simulink subsystem "inverterIn"  (R2022b)
settings: Solver=VariableStepAuto  StartTime=0.0  StopTime=10.0  RelTol=1e-3
libraries: Raptor_lib x19
settings Model: Creator=serga  LastModifiedBy=serga

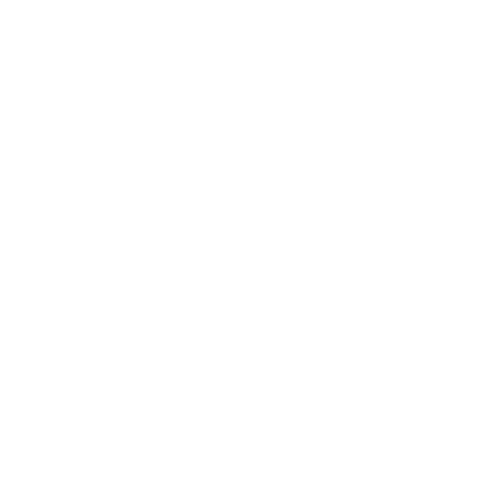
[thumbnail: Simulink's stored preview of the top-level diagram]
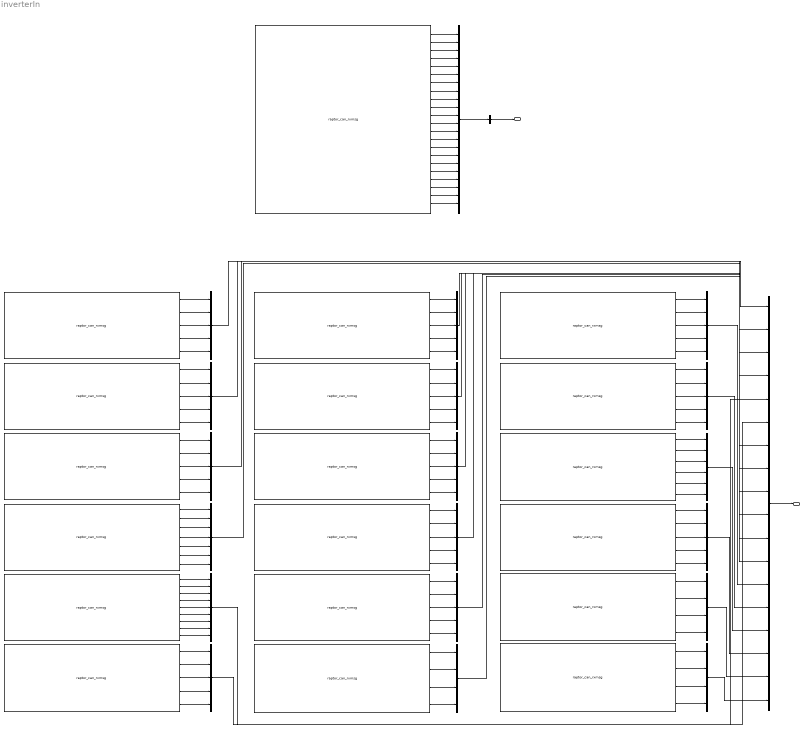
== system inverterIn ==
  note: CAN1
  note: CAN2
  Bus Creator : BusCreator  Inputs=22
  Bus Creator{1..3,6..11,13..14,16} (12 alike) : BusCreator  Inputs=5
  Bus Creator12 : BusCreator  Inputs=4
  Bus Creator15 : BusCreator  Inputs=6
  Bus Creator17 : BusCreator  Inputs=4
  Bus Creator18 : BusCreator  Inputs=4
  Bus Creator19 : BusCreator  Inputs=1
  Bus Creator20 : BusCreator  Inputs=18
  Bus Creator4 : BusCreator  Inputs=7
  Bus Creator5 : BusCreator  Inputs=9
  raptor_can_rxmsg1 : Raptor_lib/CAN/raptor_can_rxmsg  canDefinition=struct('dbcFile', 'raptor_CAN2.dbc','message', 'PM_161','comment', '','signals', {{'PM_controlBoardTemp','PM_rtd1Temp','PM_rtd2Temp','PM_rtd3Temp'}},'enabled', [ 1 1 1 1;],'scaled', [ 1 1 1 1;],'canBus', '''CAN2''','messageID', [ 161;],'idMask', [ 536870911;],'payloadMask', [],'payloadValue', [],'period', [ 0;],'mailbox', '''''','queueSize', [ 1;],'label', [ 1;],'ver', [ 2;],'showID', [ 0;],'showRaw', [ 0;],'showRawMsg', [ 0;],'useStartVals', [ 0;],'extendedId', [ 0;],'showAge', [ 1;],'useSimFunc', [ 0;],'sim_func_name', '''''','fill', [ 0;],'editID', [ 0;],'signalOrder', [ 1;],'signalAscDes', [ 1;],'msgLength', [ 8;])  canBus='CAN2'  mailbox=''  payloadMask=[]  payloadValue=[]  idMask=hex2dec('1FFFFFFF')  queueSize=1  showID=0  label=1  fill=0  id=161  showRaw=0  showAge=1  signalOrder=1  signalInfo={{struct('Name', 'PM_rtd3Temp','StartBit', [ 48;],'SignalSize', [ 16;],'ByteOrder', 'LittleEndian','ValueType', 'SIGNED','Class', 'int16','Signed', [ 1;],'Factor', [ 0.1;],'Offset', [ 0;],'Min', [ -3276.8;],'Max', [ 3276.7;],'Units', 'degC','StartVal', [ 0;],'Comment', 'RTD Input 3 (PT1000) Temperature (Gen 2 Only)','Multiplexed', [ 0;],'Multiplexor', [ 0;],'MultiplexMode_Min', [ 0;],'MultiplexMode_Max', [ 0;]),struct('Name', 'PM_rtd2Temp','StartBit', [ 32;],'SignalSize', [ 16;],'ByteOrder', 'LittleEndian','ValueType', 'SIGNED','Class', 'int16','Signed', [ 1;],'Factor', [ 0.1;],'Offset', [ 0;],'Min', [ -3276.8;],'Max', [ 3276.7;],'Units', 'degC','StartVal', [ 0;],'Comment', 'RTD Input 2 (PT1000) Temperature','Multiplexed', [ 0;],'Multiplexor', [ 0;],'MultiplexMode_Min', [ 0;],'MultiplexMode_Max', [ 0;]),struct('Name', 'PM_rtd1Temp','StartBit', [ 16;],'SignalSize', [ 16;],'ByteOrder', 'LittleEndian','ValueType', 'SIGNED','Class', 'int16','Signed', [ 1;],'Factor', [ 0.1;],'Offset', [ 0;],'Min', [ -3276.8;],'Max', [ 3276.7;],'Units', 'degC','StartVal', [ 0;],'Comment', 'RTD Input 1 (PT1000) Temperature','Multiplexed', [ 0;],'Multiplexor', [ 0;],'MultiplexMode_Min', [ 0;],'MultiplexMode_Max', [ 0;]),struct('Name', 'PM_controlBoardTemp','StartBit', [ 0;],'SignalSize', [ 16;],'ByteOrder', 'LittleEndian','ValueType', 'SIGNED','Class', 'int16','Signed', [ 1;],'Factor', [ 0.1;],'Offset', [ 0;],'Min', [ -3276.8;],'Max', [ 3276.7;],'Units', 'degC','StartVal', [ 0;],'Comment', 'Control Board Temperature','Multiplexed', [ 0;],'Multiplexor', [ 0;],'MultiplexMode_Min', [ 0;],'MultiplexMode_Max', [ 0;])}}  showRawMsg=0  useSimFunc=0  sim_func_name=''  useStartVals=0  extendedId=0
      settings: SourceProductName=Raptor
  raptor_can_rxmsg10 : Raptor_lib/CAN/raptor_can_rxmsg  canDefinition=struct('dbcFile', 'raptor_CAN2.dbc','message', 'PM_169','comment', '','signals', {{'PM_refVolt120','PM_refVolt15','PM_refVolt25','PM_refVolt50'}},'enabled', [ 1 1 1 1;],'scaled', [ 1 1 1 1;],'canBus', '''CAN2''','messageID', [ 169;],'idMask', [ 536870911;],'payloadMask', [],'payloadValue', [],'period', [ 0;],'mailbox', '''''','queueSize', [ 1;],'label', [ 1;],'ver', [ 2;],'showID', [ 0;],'showRaw', [ 0;],'showRawMsg', [ 0;],'useStartVals', [ 0;],'extendedId', [ 0;],'showAge', [ 1;],'useSimFunc', [ 0;],'sim_func_name', '''''','fill', [ 0;],'editID', [ 0;],'signalOrder', [ 1;],'signalAscDes', [ 1;],'msgLength', [ 8;])  canBus='CAN2'  mailbox=''  payloadMask=[]  payloadValue=[]  idMask=hex2dec('1FFFFFFF')  queueSize=1  showID=0  label=1  fill=0  id=169  showRaw=0  showAge=1  signalOrder=1  signalInfo={{struct('Name', 'PM_refVolt50','StartBit', [ 32;],'SignalSize', [ 16;],'ByteOrder', 'LittleEndian','ValueType', 'SIGNED','Class', 'int16','Signed', [ 1;],'Factor', [ 0.01;],'Offset', [ 0;],'Min', [ -327.68;],'Max', [ 327.67;],'Units', 'V','StartVal', [ 0;],'Comment', 'Transducer voltage','Multiplexed', [ 0;],'Multiplexor', [ 0;],'MultiplexMode_Min', [ 0;],'MultiplexMode_Max', [ 0;]),struct('Name', 'PM_refVolt25','StartBit', [ 16;],'SignalSize', [ 16;],'ByteOrder', 'LittleEndian','ValueType', 'SIGNED','Class', 'int16','Signed', [ 1;],'Factor', [ 0.01;],'Offset', [ 0;],'Min', [ -327.68;],'Max', [ 327.67;],'Units', 'V','StartVal', [ 0;],'Comment', 'Internal reference voltage','Multiplexed', [ 0;],'Multiplexor', [ 0;],'MultiplexMode_Min', [ 0;],'MultiplexMode_Max', [ 0;]),struct('Name', 'PM_refVolt15','StartBit', [ 0;],'SignalSize', [ 16;],'ByteOrder', 'LittleEndian','ValueType', 'SIGNED','Class', 'int16','Signed', [ 1;],'Factor', [ 0.01;],'Offset', [ 0;],'Min', [ -327.68;],'Max', [ 327.67;],'Units', 'V','StartVal', [ 0;],'Comment', 'Internal reference voltage','Multiplexed', [ 0;],'Multiplexor', [ 0;],'MultiplexMode_Min', [ 0;],'MultiplexMode_Max', [ 0;]),struct('Name', 'PM_refVolt120','StartBit', [ 48;],'SignalSize', [ 16;],'ByteOrder', 'LittleEndian','ValueType', 'SIGNED','Class', 'int16','Signed', [ 1;],'Factor', [ 0.01;],'Offset', [ 0;],'Min', [ -327.68;],'Max', [ 327.67;],'Units', 'V','StartVal', [ 0;],'Comment', '12V Input Voltage','Multiplexed', [ 0;],'Multiplexor', [ 0;],'MultiplexMode_Min', [ 0;],'MultiplexMode_Max', [ 0;])}}  showRawMsg=0  useSimFunc=0  sim_func_name=''  useStartVals=0  extendedId=0
      settings: SourceProductName=Raptor
  raptor_can_rxmsg11 : Raptor_lib/CAN/raptor_can_rxmsg  canDefinition=struct('dbcFile', 'raptor_CAN2.dbc','message', 'PM_171','comment', '','signals', {{'PM_postFaultHi','PM_postFaultLo','PM_runFaultHi','PM_runFaultLo'}},'enabled', [ 1 1 1 1;],'scaled', [ 1 1 1 1;],'canBus', '''CAN2''','messageID', [ 171;],'idMask', [ 536870911;],'payloadMask', [],'payloadValue', [],'period', [ 0;],'mailbox', '''''','queueSize', [ 1;],'label', [ 1;],'ver', [ 2;],'showID', [ 0;],'showRaw', [ 0;],'showRawMsg', [ 0;],'useStartVals', [ 0;],'extendedId', [ 0;],'showAge', [ 1;],'useSimFunc', [ 0;],'sim_func_name', '''''','fill', [ 0;],'editID', [ 0;],'signalOrder', [ 1;],'signalAscDes', [ 1;],'msgLength', [ 8;])  canBus='CAN2'  mailbox=''  payloadMask=[]  payloadValue=[]  idMask=hex2dec('1FFFFFFF')  queueSize=1  showID=0  label=1  fill=0  id=171  showRaw=0  showAge=1  signalOrder=1  signalInfo={{struct('Name', 'PM_runFaultLo','StartBit', [ 32;],'SignalSize', [ 16;],'ByteOrder', 'LittleEndian','ValueType', 'SIGNED','Class', 'int16','Signed', [ 1;],'Factor', [ 1;],'Offset', [ 0;],'Min', [ -32768;],'Max', [ 32767;],'Units', '','StartVal', [ 0;],'Comment', 'Each bit represents a fault. Please refer to PM100 Users Manual for details','Multiplexed', [ 0;],'Multiplexor', [ 0;],'MultiplexMode_Min', [ 0;],'MultiplexMode_Max', [ 0;]),struct('Name', 'PM_runFaultHi','StartBit', [ 48;],'SignalSize', [ 16;],'ByteOrder', 'LittleEndian','ValueType', 'SIGNED','Class', 'int16','Signed', [ 1;],'Factor', [ 1;],'Offset', [ 0;],'Min', [ -32768;],'Max', [ 32767;],'Units', '','StartVal', [ 0;],'Comment', 'Each bit represents a fault. Please refer to PM100 Users Manual for details','Multiplexed', [ 0;],'Multiplexor', [ 0;],'MultiplexMode_Min', [ 0;],'MultiplexMode_Max', [ 0;]),struct('Name', 'PM_postFaultLo','StartBit', [ 0;],'SignalSize', [ 16;],'ByteOrder', 'LittleEndian','ValueType', 'SIGNED','Class', 'int16','Signed', [ 1;],'Factor', [ 1;],'Offset', [ 0;],'Min', [ -32768;],'Max', [ 32767;],'Units', '','StartVal', [ 0;],'Comment', 'Each bit represents a fault. Please refer to PM100 Users Manual for details','Multiplexed', [ 0;],'Multiplexor', [ 0;],'MultiplexMode_Min', [ 0;],'MultiplexMode_Max', [ 0;]),struct('Name', 'PM_postFaultHi','StartBit', [ 16;],'SignalSize', [ 16;],'ByteOrder', 'LittleEndian','ValueType', 'SIGNED','Class', 'int16','Signed', [ 1;],'Factor', [ 1;],'Offset', [ 0;],'Min', [ -32768;],'Max', [ 32767;],'Units', '','StartVal', [ 0;],'Comment', 'Each bit represents a fault. Please refer to PM100 Users Manual for details','Multiplexed', [ 0;],'Multiplexor', [ 0;],'MultiplexMode_Min', [ 0;],'MultiplexMode_Max', [ 0;])}}  showRawMsg=0  useSimFunc=0  sim_func_name=''  useStartVals=0  extendedId=0
      settings: SourceProductName=Raptor
  raptor_can_rxmsg12 : Raptor_lib/CAN/raptor_can_rxmsg  canDefinition=struct('dbcFile', 'raptor_CAN2.dbc','message', 'PM_172','comment', '','signals', {{'PM_commandedTorque','PM_powerOnTimer','PM_torqueFeedback'}},'enabled', [ 1 1 1;],'scaled', [ 1 1 1;],'canBus', '''CAN2''','messageID', [ 172;],'idMask', [ 536870911;],'payloadMask', [],'payloadValue', [],'period', [ 0;],'mailbox', '''''','queueSize', [ 1;],'label', [ 1;],'ver', [ 2;],'showID', [ 0;],'showRaw', [ 0;],'showRawMsg', [ 0;],'useStartVals', [ 0;],'extendedId', [ 0;],'showAge', [ 1;],'useSimFunc', [ 0;],'sim_func_name', '''''','fill', [ 0;],'editID', [ 0;],'signalOrder', [ 1;],'signalAscDes', [ 1;],'msgLength', [ 8;])  canBus='CAN2'  mailbox=''  payloadMask=[]  payloadValue=[]  idMask=hex2dec('1FFFFFFF')  queueSize=1  showID=0  label=1  fill=0  id=172  showRaw=0  showAge=1  signalOrder=1  signalInfo={{struct('Name', 'PM_torqueFeedback','StartBit', [ 16;],'SignalSize', [ 16;],'ByteOrder', 'LittleEndian','ValueType', 'SIGNED','Class', 'int16','Signed', [ 1;],'Factor', [ 0.1;],'Offset', [ 0;],'Min', [ -3276.8;],'Max', [ 3276.7;],'Units', 'Nm','StartVal', [ 0;],'Comment', 'Estimated motor torque feedback','Multiplexed', [ 0;],'Multiplexor', [ 0;],'MultiplexMode_Min', [ 0;],'MultiplexMode_Max', [ 0;]),struct('Name', 'PM_powerOnTimer','StartBit', [ 32;],'SignalSize', [ 32;],'ByteOrder', 'LittleEndian','ValueType', 'UNSIGNED','Class', 'uint32','Signed', [ 0;],'Factor', [ 0.003;],'Offset', [ 0;],'Min', [ 0;],'Max', [ 12884800;],'Units', 'sec','StartVal', [ 0;],'Comment', 'Updated every 3 msec. This will roll over in approximately 150 days!','Multiplexed', [ 0;],'Multiplexor', [ 0;],'MultiplexMode_Min', [ 0;],'MultiplexMode_Max', [ 0;]),struct('Name', 'PM_commandedTorque','StartBit', [ 0;],'SignalSize', [ 16;],'ByteOrder', 'LittleEndian','ValueType', 'SIGNED','Class', 'int16','Signed', [ 1;],'Factor', [ 0.1;],'Offset', [ 0;],'Min', [ -3276.8;],'Max', [ 3276.7;],'Units', 'Nm','StartVal', [ 0;],'Comment', 'The commanded torque','Multiplexed', [ 0;],'Multiplexor', [ 0;],'MultiplexMode_Min', [ 0;],'MultiplexMode_Max', [ 0;])}}  showRawMsg=0  useSimFunc=0  sim_func_name=''  useStartVals=0  extendedId=0
      settings: SourceProductName=Raptor
  raptor_can_rxmsg13 : Raptor_lib/CAN/raptor_can_rxmsg  canDefinition=struct('dbcFile', 'raptor_CAN2.dbc','message', 'PM_173','comment', '','signals', {{'PM_fluxWeakeningOutput','PM_idCommand','PM_iqCommand','PM_modulationIndex'}},'enabled', [ 1 1 1 1;],'scaled', [ 1 1 1 1;],'canBus', '''CAN2''','messageID', [ 173;],'idMask', [ 536870911;],'payloadMask', [],'payloadValue', [],'period', [ 0;],'mailbox', '''''','queueSize', [ 1;],'label', [ 1;],'ver', [ 2;],'showID', [ 0;],'showRaw', [ 0;],'showRawMsg', [ 0;],'useStartVals', [ 0;],'extendedId', [ 0;],'showAge', [ 1;],'useSimFunc', [ 0;],'sim_func_name', '''''','fill', [ 0;],'editID', [ 0;],'signalOrder', [ 1;],'signalAscDes', [ 1;],'msgLength', [ 8;])  canBus='CAN2'  mailbox=''  payloadMask=[]  payloadValue=[]  idMask=hex2dec('1FFFFFFF')  queueSize=1  showID=0  label=1  fill=0  id=173  showRaw=0  showAge=1  signalOrder=1  signalInfo={{struct('Name', 'PM_modulationIndex','StartBit', [ 0;],'SignalSize', [ 16;],'ByteOrder', 'LittleEndian','ValueType', 'SIGNED','Class', 'int16','Signed', [ 1;],'Factor', [ 0.0001;],'Offset', [ 0;],'Min', [ -3.2768;],'Max', [ 3.2767;],'Units', '','StartVal', [ 0;],'Comment', 'This is the modulation index. The scale factor is x100. To get the actual modulation index divide value by 100','Multiplexed', [ 0;],'Multiplexor', [ 0;],'MultiplexMode_Min', [ 0;],'MultiplexMode_Max', [ 0;]),struct('Name', 'PM_iqCommand','StartBit', [ 48;],'SignalSize', [ 16;],'ByteOrder', 'LittleEndian','ValueType', 'SIGNED','Class', 'int16','Signed', [ 1;],'Factor', [ 0.1;],'Offset', [ 0;],'Min', [ -3276.8;],'Max', [ 3276.7;],'Units', 'A','StartVal', [ 0;],'Comment', 'The commanded Q-axis current','Multiplexed', [ 0;],'Multiplexor', [ 0;],'MultiplexMode_Min', [ 0;],'MultiplexMode_Max', [ 0;]),struct('Name', 'PM_idCommand','StartBit', [ 32;],'SignalSize', [ 16;],'ByteOrder', 'LittleEndian','ValueType', 'SIGNED','Class', 'int16','Signed', [ 1;],'Factor', [ 0.1;],'Offset', [ 0;],'Min', [ -3276.8;],'Max', [ 3276.7;],'Units', 'A','StartVal', [ 0;],'Comment', 'The commanded D-axis current','Multiplexed', [ 0;],'Multiplexor', [ 0;],'MultiplexMode_Min', [ 0;],'MultiplexMode_Max', [ 0;]),struct('Name', 'PM_fluxWeakeningOutput','StartBit', [ 16;],'SignalSize', [ 16;],'ByteOrder', 'LittleEndian','ValueType', 'SIGNED','Class', 'int16','Signed', [ 1;],'Factor', [ 0.1;],'Offset', [ 0;],'Min', [ -3276.8;],'Max', [ 3276.7;],'Units', 'A','StartVal', [ 0;],'Comment', 'This is the current output of the flux generator','Multiplexed', [ 0;],'Multiplexor', [ 0;],'MultiplexMode_Min', [ 0;],'MultiplexMode_Max', [ 0;])}}  showRawMsg=0  useSimFunc=0  sim_func_name=''  useStartVals=0  extendedId=0
      settings: SourceProductName=Raptor
  raptor_can_rxmsg14 : Raptor_lib/CAN/raptor_can_rxmsg  canDefinition=struct('dbcFile', 'raptor_CAN2.dbc','message', 'PM_174','comment', '','signals', {{'PM_datecodeMMDD','PM_datecodeYYYY','PM_projectCodeEEPVer','PM_swVersion'}},'enabled', [ 1 1 1 1;],'scaled', [ 1 1 1 1;],'canBus', '''CAN2''','messageID', [ 174;],'idMask', [ 536870911;],'payloadMask', [],'payloadValue', [],'period', [ 0;],'mailbox', '''''','queueSize', [ 1;],'label', [ 1;],'ver', [ 2;],'showID', [ 0;],'showRaw', [ 0;],'showRawMsg', [ 0;],'useStartVals', [ 0;],'extendedId', [ 0;],'showAge', [ 1;],'useSimFunc', [ 0;],'sim_func_name', '''''','fill', [ 0;],'editID', [ 0;],'signalOrder', [ 1;],'signalAscDes', [ 1;],'msgLength', [ 8;])  canBus='CAN2'  mailbox=''  payloadMask=[]  payloadValue=[]  idMask=hex2dec('1FFFFFFF')  queueSize=1  showID=0  label=1  fill=0  id=174  showRaw=0  showAge=1  signalOrder=1  signalInfo={{struct('Name', 'PM_swVersion','StartBit', [ 16;],'SignalSize', [ 16;],'ByteOrder', 'LittleEndian','ValueType', 'UNSIGNED','Class', 'uint16','Signed', [ 0;],'Factor', [ 1;],'Offset', [ 0;],'Min', [ 0;],'Max', [ 65535;],'Units', '','StartVal', [ 0;],'Comment', '','Multiplexed', [ 0;],'Multiplexor', [ 0;],'MultiplexMode_Min', [ 0;],'MultiplexMode_Max', [ 0;]),struct('Name', 'PM_projectCodeEEPVer','StartBit', [ 0;],'SignalSize', [ 16;],'ByteOrder', 'LittleEndian','ValueType', 'UNSIGNED','Class', 'uint16','Signed', [ 0;],'Factor', [ 1;],'Offset', [ 0;],'Min', [ 0;],'Max', [ 65535;],'Units', '','StartVal', [ 0;],'Comment', '','Multiplexed', [ 0;],'Multiplexor', [ 0;],'MultiplexMode_Min', [ 0;],'MultiplexMode_Max', [ 0;]),struct('Name', 'PM_datecodeYYYY','StartBit', [ 48;],'SignalSize', [ 16;],'ByteOrder', 'LittleEndian','ValueType', 'UNSIGNED','Class', 'uint16','Signed', [ 0;],'Factor', [ 1;],'Offset', [ 0;],'Min', [ 0;],'Max', [ 65535;],'Units', '','StartVal', [ 0;],'Comment', '','Multiplexed', [ 0;],'Multiplexor', [ 0;],'MultiplexMode_Min', [ 0;],'MultiplexMode_Max', [ 0;]),struct('Name', 'PM_datecodeMMDD','StartBit', [ 32;],'SignalSize', [ 16;],'ByteOrder', 'LittleEndian','ValueType', 'UNSIGNED','Class', 'uint16','Signed', [ 0;],'Factor', [ 1;],'Offset', [ 0;],'Min', [ 0;],'Max', [ 65535;],'Units', '','StartVal', [ 0;],'Comment', '','Multiplexed', [ 0;],'Multiplexor', [ 0;],'MultiplexMode_Min', [ 0;],'MultiplexMode_Max', [ 0;])}}  showRawMsg=0  useSimFunc=0  sim_func_name=''  useStartVals=0  extendedId=0
      settings: SourceProductName=Raptor
  raptor_can_rxmsg15 : Raptor_lib/CAN/raptor_can_rxmsg  canDefinition=struct('dbcFile', 'raptor_CAN2.dbc','message', 'PM_175','comment', '','signals', {{'PM_bufferRecord','PM_bufferSegment','PM_diagData1','PM_diagData2','PM_diagData3'}},'enabled', [ 1 1 1 1 1;],'scaled', [ 1 1 1 1 1;],'canBus', '''CAN2''','messageID', [ 175;],'idMask', [ 536870911;],'payloadMask', [],'payloadValue', [],'period', [ 0;],'mailbox', '''''','queueSize', [ 1;],'label', [ 1;],'ver', [ 2;],'showID', [ 0;],'showRaw', [ 0;],'showRawMsg', [ 0;],'useStartVals', [ 0;],'extendedId', [ 0;],'showAge', [ 1;],'useSimFunc', [ 0;],'sim_func_name', '''''','fill', [ 0;],'editID', [ 0;],'signalOrder', [ 1;],'signalAscDes', [ 1;],'msgLength', [ 8;])  canBus='CAN2'  mailbox=''  payloadMask=[]  payloadValue=[]  idMask=hex2dec('1FFFFFFF')  queueSize=1  showID=0  label=1  fill=0  id=175  showRaw=0  showAge=1  signalOrder=1  signalInfo={{struct('Name', 'PM_diagData3','StartBit', [ 48;],'SignalSize', [ 16;],'ByteOrder', 'LittleEndian','ValueType', 'SIGNED','Class', 'int16','Signed', [ 1;],'Factor', [ 1;],'Offset', [ 0;],'Min', [ -32768;],'Max', [ 32767;],'Units', '','StartVal', [ 0;],'Comment', '','Multiplexed', [ 0;],'Multiplexor', [ 0;],'MultiplexMode_Min', [ 0;],'MultiplexMode_Max', [ 0;]),struct('Name', 'PM_diagData2','StartBit', [ 32;],'SignalSize', [ 16;],'ByteOrder', 'LittleEndian','ValueType', 'SIGNED','Class', 'int16','Signed', [ 1;],'Factor', [ 1;],'Offset', [ 0;],'Min', [ -32768;],'Max', [ 32767;],'Units', '','StartVal', [ 0;],'Comment', '','Multiplexed', [ 0;],'Multiplexor', [ 0;],'MultiplexMode_Min', [ 0;],'MultiplexMode_Max', [ 0;]),struct('Name', 'PM_diagData1','StartBit', [ 16;],'SignalSize', [ 16;],'ByteOrder', 'LittleEndian','ValueType', 'SIGNED','Class', 'int16','Signed', [ 1;],'Factor', [ 1;],'Offset', [ 0;],'Min', [ -32768;],'Max', [ 32767;],'Units', '','StartVal', [ 0;],'Comment', '','Multiplexed', [ 0;],'Multiplexor', [ 0;],'MultiplexMode_Min', [ 0;],'MultiplexMode_Max', [ 0;]),struct('Name', 'PM_bufferSegment','StartBit', [ 8;],'SignalSize', [ 8;],'ByteOrder', 'LittleEndian','ValueType', 'UNSIGNED','Class', 'uint8','Signed', [ 0;],'Factor', [ 1;],'Offset', [ 0;],'Min', [ 0;],'Max', [ 5;],'Units', '','StartVal', [ 0;],'Comment', '','Multiplexed', [ 0;],'Multiplexor', [ 0;],'MultiplexMode_Min', [ 0;],'MultiplexMode_Max', [ 0;]),struct('Name', 'PM_bufferRecord','StartBit', [ 0;],'SignalSize', [ 8;],'ByteOrder', 'LittleEndian','ValueType', 'UNSIGNED','Class', 'uint8','Signed', [ 0;],'Factor', [ 1;],'Offset', [ 0;],'Min', [ 0;],'Max', [ 255;],'Units', '','StartVal', [ 0;],'Comment', '','Multiplexed', [ 0;],'Multiplexor', [ 0;],'MultiplexMode_Min', [ 0;],'MultiplexMode_Max', [ 0;])}}  showRawMsg=0  useSimFunc=0  sim_func_name=''  useStartVals=0  extendedId=0
      settings: SourceProductName=Raptor
  raptor_can_rxmsg16 : Raptor_lib/CAN/raptor_can_rxmsg  canDefinition=struct('dbcFile', 'raptor_CAN2.dbc','message', 'PM_176','comment', '','signals', {{'PM_fastDCBusVolt','PM_fastMotorSpeed','PM_fastTorqueCommand','PM_fastTorqueFeedback'}},'enabled', [ 1 1 1 1;],'scaled', [ 1 1 1 1;],'canBus', '''CAN2''','messageID', [ 176;],'idMask', [ 536870911;],'payloadMask', [],'payloadValue', [],'period', [ 0;],'mailbox', '''''','queueSize', [ 1;],'label', [ 1;],'ver', [ 2;],'showID', [ 0;],'showRaw', [ 0;],'showRawMsg', [ 0;],'useStartVals', [ 0;],'extendedId', [ 0;],'showAge', [ 1;],'useSimFunc', [ 0;],'sim_func_name', '''''','fill', [ 0;],'editID', [ 0;],'signalOrder', [ 1;],'signalAscDes', [ 1;],'msgLength', [ 8;])  canBus='CAN2'  mailbox=''  payloadMask=[]  payloadValue=[]  idMask=hex2dec('1FFFFFFF')  queueSize=1  showID=0  label=1  fill=0  id=176  showRaw=0  showAge=1  signalOrder=1  signalInfo={{struct('Name', 'PM_fastTorqueFeedback','StartBit', [ 16;],'SignalSize', [ 16;],'ByteOrder', 'LittleEndian','ValueType', 'SIGNED','Class', 'int16','Signed', [ 1;],'Factor', [ 0.1;],'Offset', [ 0;],'Min', [ -3276.8;],'Max', [ 3276.7;],'Units', 'Nm','StartVal', [ 0;],'Comment', 'The estimated torque','Multiplexed', [ 0;],'Multiplexor', [ 0;],'MultiplexMode_Min', [ 0;],'MultiplexMode_Max', [ 0;]),struct('Name', 'PM_fastTorqueCommand','StartBit', [ 0;],'SignalSize', [ 16;],'ByteOrder', 'LittleEndian','ValueType', 'SIGNED','Class', 'int16','Signed', [ 1;],'Factor', [ 0.1;],'Offset', [ 0;],'Min', [ -3276.8;],'Max', [ 3276.7;],'Units', 'Nm','StartVal', [ 0;],'Comment', 'The commanded torque','Multiplexed', [ 0;],'Multiplexor', [ 0;],'MultiplexMode_Min', [ 0;],'MultiplexMode_Max', [ 0;]),struct('Name', 'PM_fastMotorSpeed','StartBit', [ 32;],'SignalSize', [ 16;],'ByteOrder', 'LittleEndian','ValueType', 'SIGNED','Class', 'int16','Signed', [ 1;],'Factor', [ 1;],'Offset', [ 0;],'Min', [ -32768;],'Max', [ 32767;],'Units', 'rpm','StartVal', [ 0;],'Comment', 'Motor speed','Multiplexed', [ 0;],'Multiplexor', [ 0;],'MultiplexMode_Min', [ 0;],'MultiplexMode_Max', [ 0;]),struct('Name', 'PM_fastDCBusVolt','StartBit', [ 48;],'SignalSize', [ 16;],'ByteOrder', 'LittleEndian','ValueType', 'SIGNED','Class', 'int16','Signed', [ 1;],'Factor', [ 0.1;],'Offset', [ 0;],'Min', [ -3276.8;],'Max', [ 3276.7;],'Units', 'V','StartVal', [ 0;],'Comment', 'DC bus voltage','Multiplexed', [ 0;],'Multiplexor', [ 0;],'MultiplexMode_Min', [ 0;],'MultiplexMode_Max', [ 0;])}}  showRawMsg=0  useSimFunc=0  sim_func_name=''  useStartVals=0  extendedId=0
      settings: SourceProductName=Raptor
  raptor_can_rxmsg17 : Raptor_lib/CAN/raptor_can_rxmsg  canDefinition=struct('dbcFile', 'raptor_CAN2.dbc','message', 'PM_193','comment', '','signals', {{'PM_dataCommand','PM_parameterAddressCommand','PM_readWriteCommand'}},'enabled', [ 1 1 1;],'scaled', [ 1 1 1;],'canBus', '''CAN2''','messageID', [ 193;],'idMask', [ 536870911;],'payloadMask', [],'payloadValue', [],'period', [ 0;],'mailbox', '''''','queueSize', [ 1;],'label', [ 1;],'ver', [ 2;],'showID', [ 0;],'showRaw', [ 0;],'showRawMsg', [ 0;],'useStartVals', [ 0;],'extendedId', [ 0;],'showAge', [ 1;],'useSimFunc', [ 0;],'sim_func_name', '''''','fill', [ 0;],'editID', [ 0;],'signalOrder', [ 1;],'signalAscDes', [ 1;],'msgLength', [ 8;])  canBus='CAN2'  mailbox=''  payloadMask=[]  payloadValue=[]  idMask=hex2dec('1FFFFFFF')  queueSize=1  showID=0  label=1  fill=0  id=193  showRaw=0  showAge=1  signalOrder=1  signalInfo={{struct('Name', 'PM_readWriteCommand','StartBit', [ 16;],'SignalSize', [ 1;],'ByteOrder', 'LittleEndian','ValueType', 'UNSIGNED','Class', 'uint8','Signed', [ 0;],'Factor', [ 1;],'Offset', [ 0;],'Min', [ 0;],'Max', [ 1;],'Units', '','StartVal', [ 0;],'Comment', '0 = Read, 1 = Write','Multiplexed', [ 0;],'Multiplexor', [ 0;],'MultiplexMode_Min', [ 0;],'MultiplexMode_Max', [ 0;]),struct('Name', 'PM_parameterAddressCommand','StartBit', [ 0;],'SignalSize', [ 16;],'ByteOrder', 'LittleEndian','ValueType', 'UNSIGNED','Class', 'uint16','Signed', [ 0;],'Factor', [ 1;],'Offset', [ 0;],'Min', [ 0;],'Max', [ 65535;],'Units', '','StartVal', [ 0;],'Comment', 'Valid EEPROM Parameter CAN addresses are between 100 and 499','Multiplexed', [ 0;],'Multiplexor', [ 0;],'MultiplexMode_Min', [ 0;],'MultiplexMode_Max', [ 0;]),struct('Name', 'PM_dataCommand','StartBit', [ 32;],'SignalSize', [ 16;],'ByteOrder', 'LittleEndian','ValueType', 'SIGNED','Class', 'int16','Signed', [ 1;],'Factor', [ 1;],'Offset', [ 0;],'Min', [ -32768;],'Max', [ 32767;],'Units', '','StartVal', [ 0;],'Comment', 'All EEPROM data is 16 bits and is contained in bytes 4 and 5','Multiplexed', [ 0;],'Multiplexor', [ 0;],'MultiplexMode_Min', [ 0;],'MultiplexMode_Max', [ 0;])}}  showRawMsg=0  useSimFunc=0  sim_func_name=''  useStartVals=0  extendedId=0
      settings: SourceProductName=Raptor
  raptor_can_rxmsg18 : Raptor_lib/CAN/raptor_can_rxmsg  canDefinition=struct('dbcFile', 'raptor_CAN2.dbc','message', 'PM_194','comment', '','signals', {{'PM_dataResponse','PM_parameterAddressResponse','PM_writeSuccess'}},'enabled', [ 1 1 1;],'scaled', [ 1 1 1;],'canBus', '''CAN2''','messageID', [ 194;],'idMask', [ 536870911;],'payloadMask', [],'payloadValue', [],'period', [ 0;],'mailbox', '''''','queueSize', [ 1;],'label', [ 1;],'ver', [ 2;],'showID', [ 0;],'showRaw', [ 0;],'showRawMsg', [ 0;],'useStartVals', [ 0;],'extendedId', [ 0;],'showAge', [ 1;],'useSimFunc', [ 0;],'sim_func_name', '''''','fill', [ 0;],'editID', [ 0;],'signalOrder', [ 1;],'signalAscDes', [ 1;],'msgLength', [ 8;])  canBus='CAN2'  mailbox=''  payloadMask=[]  payloadValue=[]  idMask=hex2dec('1FFFFFFF')  queueSize=1  showID=0  label=1  fill=0  id=194  showRaw=0  showAge=1  signalOrder=1  signalInfo={{struct('Name', 'PM_writeSuccess','StartBit', [ 16;],'SignalSize', [ 1;],'ByteOrder', 'LittleEndian','ValueType', 'UNSIGNED','Class', 'uint8','Signed', [ 0;],'Factor', [ 1;],'Offset', [ 0;],'Min', [ 0;],'Max', [ 1;],'Units', '','StartVal', [ 0;],'Comment', '0 = Write Failure, 1 = Success','Multiplexed', [ 0;],'Multiplexor', [ 0;],'MultiplexMode_Min', [ 0;],'MultiplexMode_Max', [ 0;]),struct('Name', 'PM_parameterAddressResponse','StartBit', [ 0;],'SignalSize', [ 16;],'ByteOrder', 'LittleEndian','ValueType', 'UNSIGNED','Class', 'uint16','Signed', [ 0;],'Factor', [ 1;],'Offset', [ 0;],'Min', [ 0;],'Max', [ 65535;],'Units', '','StartVal', [ 0;],'Comment', 'Valid EEPROM Parameter CAN addresses are between 100 and 499','Multiplexed', [ 0;],'Multiplexor', [ 0;],'MultiplexMode_Min', [ 0;],'MultiplexMode_Max', [ 0;]),struct('Name', 'PM_dataResponse','StartBit', [ 32;],'SignalSize', [ 16;],'ByteOrder', 'LittleEndian','ValueType', 'SIGNED','Class', 'int16','Signed', [ 1;],'Factor', [ 1;],'Offset', [ 0;],'Min', [ -32768;],'Max', [ 32767;],'Units', '','StartVal', [ 0;],'Comment', 'All EEPROM data is 16 bits and is contained in bytes 4 and 5. Bytes 6 and 7 should be ignored','Multiplexed', [ 0;],'Multiplexor', [ 0;],'MultiplexMode_Min', [ 0;],'MultiplexMode_Max', [ 0;])}}  showRawMsg=0  useSimFunc=0  sim_func_name=''  useStartVals=0  extendedId=0
      settings: SourceProductName=Raptor
  raptor_can_rxmsg19 : Raptor_lib/CAN/raptor_can_rxmsg  canDefinition=struct('dbcFile', 'raptor_CAN1.dbc','message', 'PM_170','comment', '','signals', {{'PM_bmsActive','PM_bmsTorqueLimiting','PM_counterMsg170','PM_directionCommand','PM_inverterCommandMode','PM_inverterDischargeMode','PM_inverterEnableLockout','PM_inverterEnableState','PM_inverterRunMode','PM_inverterState','PM_lowSpeedLimiting','PM_maxSpeedLimiting','PM_pwmFrequency','PM_relayStatus1','PM_relayStatus2','PM_relayStatus3','PM_relayStatus4','PM_relayStatus5','PM_relayStatus6','PM_startModeActive','PM_vsmState'}},'enabled', [ 1 1 1 1 1 1 1 1 1 1 1 1 1 1 1 1 1 1 1 1 1;],'scaled', [ 1 1 1 1 1 1 1 1 1 1 1 1 1 1 1 1 1 1 1 1 1;],'canBus', '''CAN1''','messageID', [ 170;],'idMask', [ 536870911;],'payloadMask', [],'payloadValue', [],'period', [ 0;],'mailbox', '''''','queueSize', [ 1;],'label', [ 1;],'ver', [ 2;],'showID', [ 0;],'showRaw', [ 0;],'showRawMsg', [ 0;],'useStartVals', [ 0;],'extendedId', [ 0;],'showAge', [ 1;],'useSimFunc', [ 0;],'sim_func_name', '''''','fill', [ 0;],'editID', [ 0;],'signalOrder', [ 1;],'signalAscDes', [ 1;],'msgLength', [ 8;])  canBus='CAN1'  mailbox=''  payloadMask=[]  payloadValue=[]  idMask=hex2dec('1FFFFFFF')  queueSize=1  showID=0  label=1  fill=0  id=170  showRaw=0  showAge=1  signalOrder=1  signalInfo={{struct('Name', 'PM_vsmState','StartBit', [ 0;],'SignalSize', [ 8;],'ByteOrder', 'LittleEndian','ValueType', 'UNSIGNED','Class', 'uint8','Signed', [ 0;],'Factor', [ 1;],'Offset', [ 0;],'Min', [ 0;],'Max', [ 15;],'Units', '','StartVal', [ 0;],'Comment', 'Different states for the vehicle state machine','Multiplexed', [ 0;],'Multiplexor', [ 0;],'MultiplexMode_Min', [ 0;],'MultiplexMode_Max', [ 0;]),struct('Name', 'PM_startModeActive','StartBit', [ 54;],'SignalSize', [ 1;],'ByteOrder', 'LittleEndian','ValueType', 'UNSIGNED','Class', 'uint8','Signed', [ 0;],'Factor', [ 1;],'Offset', [ 0;],'Min', [ 0;],'Max', [ 1;],'Units', '','StartVal', [ 0;],'Comment', 'If in Key Switch Mode 1, indicates status of Start input being applied. 0 = Not Active, 1 = Active','Multiplexed', [ 0;],'Multiplexor', [ 0;],'MultiplexMode_Min', [ 0;],'MultiplexMode_Max', [ 0;]),struct('Name', 'PM_relayStatus6','StartBit', [ 29;],'SignalSize', [ 1;],'ByteOrder', 'LittleEndian','ValueType', 'UNSIGNED','Class', 'uint8','Signed', [ 0;],'Factor', [ 1;],'Offset', [ 0;],'Min', [ 0;],'Max', [ 1;],'Units', '','StartVal', [ 0;],'Comment', '0 = OFF, 1 = ON','Multiplexed', [ 0;],'Multiplexor', [ 0;],'MultiplexMode_Min', [ 0;],'MultiplexMode_Max', [ 0;]),struct('Name', 'PM_relayStatus5','StartBit', [ 28;],'SignalSize', [ 1;],'ByteOrder', 'LittleEndian','ValueType', 'UNSIGNED','Class', 'uint8','Signed', [ 0;],'Factor', [ 1;],'Offset', [ 0;],'Min', [ 0;],'Max', [ 1;],'Units', '','StartVal', [ 0;],'Comment', '0 = OFF, 1 = ON','Multiplexed', [ 0;],'Multiplexor', [ 0;],'MultiplexMode_Min', [ 0;],'MultiplexMode_Max', [ 0;]),struct('Name', 'PM_relayStatus4','StartBit', [ 27;],'SignalSize', [ 1;],'ByteOrder', 'LittleEndian','ValueType', 'UNSIGNED','Class', 'uint8','Signed', [ 0;],'Factor', [ 1;],'Offset', [ 0;],'Min', [ 0;],'Max', [ 1;],'Units', '','StartVal', [ 0;],'Comment', '0 = OFF, 1 = ON','Multiplexed', [ 0;],'Multiplexor', [ 0;],'MultiplexMode_Min', [ 0;],'MultiplexMode_Max', [ 0;]),struct('Name', 'PM_relayStatus3','StartBit', [ 26;],'SignalSize', [ 1;],'ByteOrder', 'LittleEndian','ValueType', 'UNSIGNED','Class', 'uint8','Signed', [ 0;],'Factor', [ 1;],'Offset', [ 0;],'Min', [ 0;],'Max', [ 1;],'Units', '','StartVal', [ 0;],'Comment', '0 = OFF, 1 = ON','Multiplexed', [ 0;],'Multiplexor', [ 0;],'MultiplexMode_Min', [ 0;],'MultiplexMode_Max', [ 0;]),struct('Name', 'PM_relayStatus2','StartBit', [ 25;],'SignalSize', [ 1;],'ByteOrder', 'LittleEndian','ValueType', 'UNSIGNED','Class', 'uint8','Signed', [ 0;],'Factor', [ 1;],'Offset', [ 0;],'Min', [ 0;],'Max', [ 1;],'Units', '','StartVal', [ 0;],'Comment', '0 = OFF, 1 = ON','Multiplexed', [ 0;],'Multiplexor', [ 0;],'MultiplexMode_Min', [ 0;],'MultiplexMode_Max', [ 0;]),struct('Name', 'PM_relayStatus1','StartBit', [ 24;],'SignalSize', [ 1;],'ByteOrder', 'LittleEndian','ValueType', 'UNSIGNED','Class', 'uint8','Signed', [ 0;],'Factor', [ 1;],'Offset', [ 0;],'Min', [ 0;],'Max', [ 1;],'Units', '','StartVal', [ 0;],'Comment', '0 = OFF, 1 = ON','Multiplexed', [ 0;],'Multiplexor', [ 0;],'MultiplexMode_Min', [ 0;],'MultiplexMode_Max', [ 0;]),struct('Name', 'PM_pwmFrequency','StartBit', [ 8;],'SignalSize', [ 8;],'ByteOrder', 'LittleEndian','ValueType', 'UNSIGNED','Class', 'uint8','Signed', [ 0;],'Factor', [ 1;],'Offset', [ 0;],'Min', [ 0;],'Max', [ 255;],'Units', 'kHz','StartVal', [ 0;],'Comment', 'The inverter PWM frequency','Multiplexed', [ 0;],'Multiplexor', [ 0;],'MultiplexMode_Min', [ 0;],'MultiplexMode_Max', [ 0;]),struct('Name', 'PM_maxSpeedLimiting','StartBit', [ 59;],'SignalSize', [ 1;],'ByteOrder', 'LittleEndian','ValueType', 'UNSIGNED','Class', 'uint8','Signed', [ 0;],'Factor', [ 1;],'Offset', [ 0;],'Min', [ 0;],'Max', [ 1;],'Units', '','StartVal', [ 0;],'Comment', '0 = Not Limiting, 1 = Torque Limiting due to Maximum Speed','Multiplexed', [ 0;],'Multiplexor', [ 0;],'MultiplexMode_Min', [ 0;],'MultiplexMode_Max', [ 0;]),struct('Name', 'PM_lowSpeedLimiting','StartBit', [ 61;],'SignalSize', [ 1;],'ByteOrder', 'LittleEndian','ValueType', 'UNSIGNED','Class', 'uint8','Signed', [ 0;],'Factor', [ 1;],'Offset', [ 0;],'Min', [ 0;],'Max', [ 1;],'Units', '','StartVal', [ 0;],'Comment', '0 = Not Limiting, 1 = Current Limiting due to Low Motor Speed','Multiplexed', [ 0;],'Multiplexor', [ 0;],'MultiplexMode_Min', [ 0;],'MultiplexMode_Max', [ 0;]),struct('Name', 'PM_inverterState','StartBit', [ 16;],'SignalSize', [ 8;],'ByteOrder', 'LittleEndian','ValueType', 'UNSIGNED','Class', 'uint8','Signed', [ 0;],'Factor', [ 1;],'Offset', [ 0;],'Min', [ 0;],'Max', [ 255;],'Units', '','StartVal', [ 0;],'Comment', 'Different states for the inverter machine state','Multiplexed', [ 0;],'Multiplexor', [ 0;],'MultiplexMode_Min', [ 0;],'MultiplexMode_Max', [ 0;]),struct('Name', 'PM_inverterRunMode','StartBit', [ 32;],'SignalSize', [ 1;],'ByteOrder', 'LittleEndian','ValueType', 'UNSIGNED','Class', 'uint8','Signed', [ 0;],'Factor', [ 1;],'Offset', [ 0;],'Min', [ 0;],'Max', [ 1;],'Units', '','StartVal', [ 0;],'Comment', '0 = Torque Mode, 1 = Speed Mode','Multiplexed', [ 0;],'Multiplexor', [ 0;],'MultiplexMode_Min', [ 0;],'MultiplexMode_Max', [ 0;]),struct('Name', 'PM_inverterEnableState','StartBit', [ 48;],'SignalSize', [ 1;],'ByteOrder', 'LittleEndian','ValueType', 'UNSIGNED','Class', 'uint8','Signed', [ 0;],'Factor', [ 1;],'Offset', [ 0;],'Min', [ 0;],'Max', [ 1;],'Units', '','StartVal', [ 0;],'Comment', '0 = Inverter Disabled, 1 = Inverter Enabled','Multiplexed', [ 0;],'Multiplexor', [ 0;],'MultiplexMode_Min', [ 0;],'MultiplexMode_Max', [ 0;]),struct('Name', 'PM_inverterEnableLockout','StartBit', [ 55;],'SignalSize', [ 1;],'ByteOrder', 'LittleEndian','ValueType', 'UNSIGNED','Class', 'uint8','Signed', [ 0;],'Factor', [ 1;],'Offset', [ 0;],'Min', [ 0;],'Max', [ 1;],'Units', '','StartVal', [ 0;],'Comment', '0 = Lockout Disabled, 1 = Lockout Enabled','Multiplexed', [ 0;],'Multiplexor', [ 0;],'MultiplexMode_Min', [ 0;],'MultiplexMode_Max', [ 0;]),struct('Name', 'PM_inverterDischargeMode','StartBit', [ 37;],'SignalSize', [ 3;],'ByteOrder', 'LittleEndian','ValueType', 'UNSIGNED','Class', 'uint8','Signed', [ 0;],'Factor', [ 1;],'Offset', [ 0;],'Min', [ 0;],'Max', [ 7;],'Units', '','StartVal', [ 0;],'Comment', '0 = Disabled, 1 = Enabled, 2 = Speed Check, 3 = Active, 4 = Complete','Multiplexed', [ 0;],'Multiplexor', [ 0;],'MultiplexMode_Min', [ 0;],'MultiplexMode_Max', [ 0;]),struct('Name', 'PM_inverterCommandMode','StartBit', [ 40;],'SignalSize', [ 1;],'ByteOrder', 'LittleEndian','ValueType', 'UNSIGNED','Class', 'uint8','Signed', [ 0;],'Factor', [ 1;],'Offset', [ 0;],'Min', [ 0;],'Max', [ 1;],'Units', '','StartVal', [ 0;],'Comment', '0 = CAN Mode, 1 = VSM Mode','Multiplexed', [ 0;],'Multiplexor', [ 0;],'MultiplexMode_Min', [ 0;],'MultiplexMode_Max', [ 0;]),struct('Name', 'PM_directionCommand','StartBit', [ 56;],'SignalSize', [ 1;],'ByteOrder', 'LittleEndian','ValueType', 'UNSIGNED','Class', 'uint8','Signed', [ 0;],'Factor', [ 1;],'Offset', [ 0;],'Min', [ 0;],'Max', [ 1;],'Units', '','StartVal', [ 0;],'Comment', '1 = Forward, 0 = `Reverse` if inverter enabled & `Stopped` if inverter is disabled','Multiplexed', [ 0;],'Multiplexor', [ 0;],'MultiplexMode_Min', [ 0;],'MultiplexMode_Max', [ 0;]),struct('Name', 'PM_counterMsg170','StartBit', [ 44;],'SignalSize', [ 4;],'ByteOrder', 'LittleEndian','ValueType', 'UNSIGNED','Class', 'uint8','Signed', [ 0;],'Factor', [ 1;],'Offset', [ 0;],'Min', [ 0;],'Max', [ 15;],'Units', '','StartVal', [ 0;],'Comment', 'Counter Message 170','Multiplexed', [ 0;],'Multiplexor', [ 0;],'MultiplexMode_Min', [ 0;],'MultiplexMode_Max', [ 0;]),struct('Name', 'PM_bmsTorqueLimiting','StartBit', [ 58;],'SignalSize', [ 1;],'ByteOrder', 'LittleEndian','ValueType', 'UNSIGNED','Class', 'uint8','Signed', [ 0;],'Factor', [ 1;],'Offset', [ 0;],'Min', [ 0;],'Max', [ 1;],'Units', '','StartVal', [ 0;],'Comment', '0 = Not Limiting, 1 = Limiting','Multiplexed', [ 0;],'Multiplexor', [ 0;],'MultiplexMode_Min', [ 0;],'MultiplexMode_Max', [ 0;]),struct('Name', 'PM_bmsActive','StartBit', [ 57;],'SignalSize', [ 1;],'ByteOrder', 'LittleEndian','ValueType', 'UNSIGNED','Class', 'uint8','Signed', [ 0;],'Factor', [ 1;],'Offset', [ 0;],'Min', [ 0;],'Max', [ 1;],'Units', '','StartVal', [ 0;],'Comment', '0 = BMS Not Active, 1 = BMS Active','Multiplexed', [ 0;],'Multiplexor', [ 0;],'MultiplexMode_Min', [ 0;],'MultiplexMode_Max', [ 0;])}}  showRawMsg=0  useSimFunc=0  sim_func_name=''  useStartVals=0  extendedId=0
      settings: SourceProductName=Raptor
  raptor_can_rxmsg2 : Raptor_lib/CAN/raptor_can_rxmsg  canDefinition=struct('dbcFile', 'raptor_CAN2.dbc','message', 'PM_160','comment', '','signals', {{'PM_gateDriverBoard','PM_moduleATemp','PM_moduleBTemp','PM_moduleCTemp'}},'enabled', [ 1 1 1 1;],'scaled', [ 1 1 1 1;],'canBus', '''CAN2''','messageID', [ 160;],'idMask', [ 536870911;],'payloadMask', [],'payloadValue', [],'period', [ 0;],'mailbox', '''''','queueSize', [ 1;],'label', [ 1;],'ver', [ 2;],'showID', [ 0;],'showRaw', [ 0;],'showRawMsg', [ 0;],'useStartVals', [ 0;],'extendedId', [ 0;],'showAge', [ 1;],'useSimFunc', [ 0;],'sim_func_name', '''''','fill', [ 0;],'editID', [ 0;],'signalOrder', [ 1;],'signalAscDes', [ 1;],'msgLength', [ 8;])  canBus='CAN2'  mailbox=''  payloadMask=[]  payloadValue=[]  idMask=hex2dec('1FFFFFFF')  queueSize=1  showID=0  label=1  fill=0  id=160  showRaw=0  showAge=1  signalOrder=1  signalInfo={{struct('Name', 'PM_moduleCTemp','StartBit', [ 32;],'SignalSize', [ 16;],'ByteOrder', 'LittleEndian','ValueType', 'SIGNED','Class', 'int16','Signed', [ 1;],'Factor', [ 0.1;],'Offset', [ 0;],'Min', [ -3276.8;],'Max', [ 3276.7;],'Units', 'degC','StartVal', [ 0;],'Comment', 'IGBT Module C Temperature','Multiplexed', [ 0;],'Multiplexor', [ 0;],'MultiplexMode_Min', [ 0;],'MultiplexMode_Max', [ 0;]),struct('Name', 'PM_moduleBTemp','StartBit', [ 16;],'SignalSize', [ 16;],'ByteOrder', 'LittleEndian','ValueType', 'SIGNED','Class', 'int16','Signed', [ 1;],'Factor', [ 0.1;],'Offset', [ 0;],'Min', [ -3276.8;],'Max', [ 3276.7;],'Units', 'degC','StartVal', [ 0;],'Comment', 'IGBT Module B Temperature','Multiplexed', [ 0;],'Multiplexor', [ 0;],'MultiplexMode_Min', [ 0;],'MultiplexMode_Max', [ 0;]),struct('Name', 'PM_moduleATemp','StartBit', [ 0;],'SignalSize', [ 16;],'ByteOrder', 'LittleEndian','ValueType', 'SIGNED','Class', 'int16','Signed', [ 1;],'Factor', [ 0.1;],'Offset', [ 0;],'Min', [ -3276.8;],'Max', [ 3276.7;],'Units', 'degC','StartVal', [ 0;],'Comment', 'IGBT Module A Temperature','Multiplexed', [ 0;],'Multiplexor', [ 0;],'MultiplexMode_Min', [ 0;],'MultiplexMode_Max', [ 0;]),struct('Name', 'PM_gateDriverBoard','StartBit', [ 48;],'SignalSize', [ 16;],'ByteOrder', 'LittleEndian','ValueType', 'SIGNED','Class', 'int16','Signed', [ 1;],'Factor', [ 0.1;],'Offset', [ 0;],'Min', [ -3276.8;],'Max', [ 3276.7;],'Units', 'degC','StartVal', [ 0;],'Comment', 'Gate Driver Board Temperature','Multiplexed', [ 0;],'Multiplexor', [ 0;],'MultiplexMode_Min', [ 0;],'MultiplexMode_Max', [ 0;])}}  showRawMsg=0  useSimFunc=0  sim_func_name=''  useStartVals=0  extendedId=0
      settings: SourceProductName=Raptor
  raptor_can_rxmsg3 : Raptor_lib/CAN/raptor_can_rxmsg  canDefinition=struct('dbcFile', 'raptor_CAN2.dbc','message', 'PM_162','comment', '','signals', {{'PM_motorTemp','PM_rtd4Temp','PM_rtd5Temp','PM_torqueShudder'}},'enabled', [ 1 1 1 1;],'scaled', [ 1 1 1 1;],'canBus', '''CAN2''','messageID', [ 162;],'idMask', [ 536870911;],'payloadMask', [],'payloadValue', [],'period', [ 0;],'mailbox', '''''','queueSize', [ 1;],'label', [ 1;],'ver', [ 2;],'showID', [ 0;],'showRaw', [ 0;],'showRawMsg', [ 0;],'useStartVals', [ 0;],'extendedId', [ 0;],'showAge', [ 1;],'useSimFunc', [ 0;],'sim_func_name', '''''','fill', [ 0;],'editID', [ 0;],'signalOrder', [ 1;],'signalAscDes', [ 1;],'msgLength', [ 8;])  canBus='CAN2'  mailbox=''  payloadMask=[]  payloadValue=[]  idMask=hex2dec('1FFFFFFF')  queueSize=1  showID=0  label=1  fill=0  id=162  showRaw=0  showAge=1  signalOrder=1  signalInfo={{struct('Name', 'PM_torqueShudder','StartBit', [ 48;],'SignalSize', [ 16;],'ByteOrder', 'LittleEndian','ValueType', 'SIGNED','Class', 'int16','Signed', [ 1;],'Factor', [ 0.1;],'Offset', [ 0;],'Min', [ -3276.8;],'Max', [ 3276.7;],'Units', 'Nm','StartVal', [ 0;],'Comment', 'Shudder Compensation Value of Torque','Multiplexed', [ 0;],'Multiplexor', [ 0;],'MultiplexMode_Min', [ 0;],'MultiplexMode_Max', [ 0;]),struct('Name', 'PM_rtd5Temp','StartBit', [ 16;],'SignalSize', [ 16;],'ByteOrder', 'LittleEndian','ValueType', 'SIGNED','Class', 'int16','Signed', [ 1;],'Factor', [ 0.1;],'Offset', [ 0;],'Min', [ -3276.8;],'Max', [ 3276.7;],'Units', 'degC','StartVal', [ 0;],'Comment', 'RTD Input 5 (PT1000) Temperature (Gen 2 Only)','Multiplexed', [ 0;],'Multiplexor', [ 0;],'MultiplexMode_Min', [ 0;],'MultiplexMode_Max', [ 0;]),struct('Name', 'PM_rtd4Temp','StartBit', [ 0;],'SignalSize', [ 16;],'ByteOrder', 'LittleEndian','ValueType', 'SIGNED','Class', 'int16','Signed', [ 1;],'Factor', [ 0.1;],'Offset', [ 0;],'Min', [ -3276.8;],'Max', [ 3276.7;],'Units', 'degC','StartVal', [ 0;],'Comment', 'RTD Input 4 (PT1000) Temperature (Gen 2 Only)','Multiplexed', [ 0;],'Multiplexor', [ 0;],'MultiplexMode_Min', [ 0;],'MultiplexMode_Max', [ 0;]),struct('Name', 'PM_motorTemp','StartBit', [ 32;],'SignalSize', [ 16;],'ByteOrder', 'LittleEndian','ValueType', 'SIGNED','Class', 'int16','Signed', [ 1;],'Factor', [ 0.1;],'Offset', [ 0;],'Min', [ -3276.8;],'Max', [ 3276.7;],'Units', 'degC','StartVal', [ 0;],'Comment', 'Motor Temperature Sensor','Multiplexed', [ 0;],'Multiplexor', [ 0;],'MultiplexMode_Min', [ 0;],'MultiplexMode_Max', [ 0;])}}  showRawMsg=0  useSimFunc=0  sim_func_name=''  useStartVals=0  extendedId=0
      settings: SourceProductName=Raptor
  raptor_can_rxmsg4 : Raptor_lib/CAN/raptor_can_rxmsg  canDefinition=struct('dbcFile', 'raptor_CAN2.dbc','message', 'PM_163','comment', '','signals', {{'PM_analogInputVolt1','PM_analogInputVolt2','PM_analogInputVolt3','PM_analogInputVolt4','PM_analogInputVolt5','PM_analogInputVolt6'}},'enabled', [ 1 1 1 1 1 1;],'scaled', [ 1 1 1 1 1 1;],'canBus', '''CAN2''','messageID', [ 163;],'idMask', [ 536870911;],'payloadMask', [],'payloadValue', [],'period', [ 0;],'mailbox', '''''','queueSize', [ 1;],'label', [ 1;],'ver', [ 2;],'showID', [ 0;],'showRaw', [ 0;],'showRawMsg', [ 0;],'useStartVals', [ 0;],'extendedId', [ 0;],'showAge', [ 1;],'useSimFunc', [ 0;],'sim_func_name', '''''','fill', [ 0;],'editID', [ 0;],'signalOrder', [ 1;],'signalAscDes', [ 1;],'msgLength', [ 8;])  canBus='CAN2'  mailbox=''  payloadMask=[]  payloadValue=[]  idMask=hex2dec('1FFFFFFF')  queueSize=1  showID=0  label=1  fill=0  id=163  showRaw=0  showAge=1  signalOrder=1  signalInfo={{struct('Name', 'PM_analogInputVolt6','StartBit', [ 52;],'SignalSize', [ 10;],'ByteOrder', 'LittleEndian','ValueType', 'UNSIGNED','Class', 'uint16','Signed', [ 0;],'Factor', [ 0.01;],'Offset', [ 0;],'Min', [ 0;],'Max', [ 10.23;],'Units', 'V','StartVal', [ 0;],'Comment', 'Voltage on Analog Input #6','Multiplexed', [ 0;],'Multiplexor', [ 0;],'MultiplexMode_Min', [ 0;],'MultiplexMode_Max', [ 0;]),struct('Name', 'PM_analogInputVolt5','StartBit', [ 42;],'SignalSize', [ 10;],'ByteOrder', 'LittleEndian','ValueType', 'UNSIGNED','Class', 'uint16','Signed', [ 0;],'Factor', [ 0.01;],'Offset', [ 0;],'Min', [ 0;],'Max', [ 10.23;],'Units', 'V','StartVal', [ 0;],'Comment', 'Voltage on Analog Input #5','Multiplexed', [ 0;],'Multiplexor', [ 0;],'MultiplexMode_Min', [ 0;],'MultiplexMode_Max', [ 0;]),struct('Name', 'PM_analogInputVolt4','StartBit', [ 32;],'SignalSize', [ 10;],'ByteOrder', 'LittleEndian','ValueType', 'UNSIGNED','Class', 'uint16','Signed', [ 0;],'Factor', [ 0.01;],'Offset', [ 0;],'Min', [ 0;],'Max', [ 10.23;],'Units', 'V','StartVal', [ 0;],'Comment', 'Voltage on Analog Input #4','Multiplexed', [ 0;],'Multiplexor', [ 0;],'MultiplexMode_Min', [ 0;],'MultiplexMode_Max', [ 0;]),struct('Name', 'PM_analogInputVolt3','StartBit', [ 20;],'SignalSize', [ 10;],'ByteOrder', 'LittleEndian','ValueType', 'UNSIGNED','Class', 'uint16','Signed', [ 0;],'Factor', [ 0.01;],'Offset', [ 0;],'Min', [ 0;],'Max', [ 10.23;],'Units', 'V','StartVal', [ 0;],'Comment', 'Voltage on Analog Input #3','Multiplexed', [ 0;],'Multiplexor', [ 0;],'MultiplexMode_Min', [ 0;],'MultiplexMode_Max', [ 0;]),struct('Name', 'PM_analogInputVolt2','StartBit', [ 10;],'SignalSize', [ 10;],'ByteOrder', 'LittleEndian','ValueType', 'UNSIGNED','Class', 'uint16','Signed', [ 0;],'Factor', [ 0.01;],'Offset', [ 0;],'Min', [ 0;],'Max', [ 10.23;],'Units', 'V','StartVal', [ 0;],'Comment', 'Voltage on Analog Input #2','Multiplexed', [ 0;],'Multiplexor', [ 0;],'MultiplexMode_Min', [ 0;],'MultiplexMode_Max', [ 0;]),struct('Name', 'PM_analogInputVolt1','StartBit', [ 0;],'SignalSize', [ 10;],'ByteOrder', 'LittleEndian','ValueType', 'UNSIGNED','Class', 'uint16','Signed', [ 0;],'Factor', [ 0.01;],'Offset', [ 0;],'Min', [ 0;],'Max', [ 10.23;],'Units', 'V','StartVal', [ 0;],'Comment', 'Voltage on Analog Input #1','Multiplexed', [ 0;],'Multiplexor', [ 0;],'MultiplexMode_Min', [ 0;],'MultiplexMode_Max', [ 0;])}}  showRawMsg=0  useSimFunc=0  sim_func_name=''  useStartVals=0  extendedId=0
      settings: SourceProductName=Raptor
  raptor_can_rxmsg5 : Raptor_lib/CAN/raptor_can_rxmsg  canDefinition=struct('dbcFile', 'raptor_CAN2.dbc','message', 'PM_164','comment', '','signals', {{'PM_digitalInputStatus1','PM_digitalInputStatus2','PM_digitalInputStatus3','PM_digitalInputStatus4','PM_digitalInputStatus5','PM_digitalInputStatus6','PM_digitalInputStatus7','PM_digitalInputStatus8'}},'enabled', [ 1 1 1 1 1 1 1 1;],'scaled', [ 1 1 1 1 1 1 1 1;],'canBus', '''CAN2''','messageID', [ 164;],'idMask', [ 536870911;],'payloadMask', [],'payloadValue', [],'period', [ 0;],'mailbox', '''''','queueSize', [ 1;],'label', [ 1;],'ver', [ 2;],'showID', [ 0;],'showRaw', [ 0;],'showRawMsg', [ 0;],'useStartVals', [ 0;],'extendedId', [ 0;],'showAge', [ 1;],'useSimFunc', [ 0;],'sim_func_name', '''''','fill', [ 0;],'editID', [ 0;],'signalOrder', [ 1;],'signalAscDes', [ 1;],'msgLength', [ 8;])  canBus='CAN2'  mailbox=''  payloadMask=[]  payloadValue=[]  idMask=hex2dec('1FFFFFFF')  queueSize=1  showID=0  label=1  fill=0  id=164  showRaw=0  showAge=1  signalOrder=1  signalInfo={{struct('Name', 'PM_digitalInputStatus8','StartBit', [ 56;],'SignalSize', [ 1;],'ByteOrder', 'LittleEndian','ValueType', 'UNSIGNED','Class', 'uint8','Signed', [ 0;],'Factor', [ 1;],'Offset', [ 0;],'Min', [ 0;],'Max', [ 1;],'Units', '','StartVal', [ 0;],'Comment', 'Status of Digital Input #8','Multiplexed', [ 0;],'Multiplexor', [ 0;],'MultiplexMode_Min', [ 0;],'MultiplexMode_Max', [ 0;]),struct('Name', 'PM_digitalInputStatus7','StartBit', [ 48;],'SignalSize', [ 1;],'ByteOrder', 'LittleEndian','ValueType', 'UNSIGNED','Class', 'uint8','Signed', [ 0;],'Factor', [ 1;],'Offset', [ 0;],'Min', [ 0;],'Max', [ 1;],'Units', '','StartVal', [ 0;],'Comment', 'Status of Digital Input #7','Multiplexed', [ 0;],'Multiplexor', [ 0;],'MultiplexMode_Min', [ 0;],'MultiplexMode_Max', [ 0;]),struct('Name', 'PM_digitalInputStatus6','StartBit', [ 40;],'SignalSize', [ 1;],'ByteOrder', 'LittleEndian','ValueType', 'UNSIGNED','Class', 'uint8','Signed', [ 0;],'Factor', [ 1;],'Offset', [ 0;],'Min', [ 0;],'Max', [ 1;],'Units', '','StartVal', [ 0;],'Comment', 'Status of Digital Input #6','Multiplexed', [ 0;],'Multiplexor', [ 0;],'MultiplexMode_Min', [ 0;],'MultiplexMode_Max', [ 0;]),struct('Name', 'PM_digitalInputStatus5','StartBit', [ 32;],'SignalSize', [ 1;],'ByteOrder', 'LittleEndian','ValueType', 'UNSIGNED','Class', 'uint8','Signed', [ 0;],'Factor', [ 1;],'Offset', [ 0;],'Min', [ 0;],'Max', [ 1;],'Units', '','StartVal', [ 0;],'Comment', 'Status of Digital Input #5','Multiplexed', [ 0;],'Multiplexor', [ 0;],'MultiplexMode_Min', [ 0;],'MultiplexMode_Max', [ 0;]),struct('Name', 'PM_digitalInputStatus4','StartBit', [ 24;],'SignalSize', [ 1;],'ByteOrder', 'LittleEndian','ValueType', 'UNSIGNED','Class', 'uint8','Signed', [ 0;],'Factor', [ 1;],'Offset', [ 0;],'Min', [ 0;],'Max', [ 1;],'Units', '','StartVal', [ 0;],'Comment', 'Status of Digital Input #4','Multiplexed', [ 0;],'Multiplexor', [ 0;],'MultiplexMode_Min', [ 0;],'MultiplexMode_Max', [ 0;]),struct('Name', 'PM_digitalInputStatus3','StartBit', [ 16;],'SignalSize', [ 1;],'ByteOrder', 'LittleEndian','ValueType', 'UNSIGNED','Class', 'uint8','Signed', [ 0;],'Factor', [ 1;],'Offset', [ 0;],'Min', [ 0;],'Max', [ 1;],'Units', '','StartVal', [ 0;],'Comment', 'Status of Digital Input #3','Multiplexed', [ 0;],'Multiplexor', [ 0;],'MultiplexMode_Min', [ 0;],'MultiplexMode_Max', [ 0;]),struct('Name', 'PM_digitalInputStatus2','StartBit', [ 8;],'SignalSize', [ 1;],'ByteOrder', 'LittleEndian','ValueType', 'UNSIGNED','Class', 'uint8','Signed', [ 0;],'Factor', [ 1;],'Offset', [ 0;],'Min', [ 0;],'Max', [ 1;],'Units', '','StartVal', [ 0;],'Comment', 'Status of Digital Input #2','Multiplexed', [ 0;],'Multiplexor', [ 0;],'MultiplexMode_Min', [ 0;],'MultiplexMode_Max', [ 0;]),struct('Name', 'PM_digitalInputStatus1','StartBit', [ 0;],'SignalSize', [ 1;],'ByteOrder', 'LittleEndian','ValueType', 'UNSIGNED','Class', 'uint8','Signed', [ 0;],'Factor', [ 1;],'Offset', [ 0;],'Min', [ 0;],'Max', [ 1;],'Units', '','StartVal', [ 0;],'Comment', 'Status of Digital Input #1','Multiplexed', [ 0;],'Multiplexor', [ 0;],'MultiplexMode_Min', [ 0;],'MultiplexMode_Max', [ 0;])}}  showRawMsg=0  useSimFunc=0  sim_func_name=''  useStartVals=0  extendedId=0
      settings: SourceProductName=Raptor
  raptor_can_rxmsg6 : Raptor_lib/CAN/raptor_can_rxmsg  canDefinition=struct('dbcFile', 'raptor_CAN2.dbc','message', 'PM_165','comment', '','signals', {{'PM_deltaResolverFiltered','PM_electricalMotorAngle','PM_electricalOutputFrequency','PM_motorSpeed'}},'enabled', [ 1 1 1 1;],'scaled', [ 1 1 1 1;],'canBus', '''CAN2''','messageID', [ 165;],'idMask', [ 536870911;],'payloadMask', [],'payloadValue', [],'period', [ 0;],'mailbox', '''''','queueSize', [ 1;],'label', [ 1;],'ver', [ 2;],'showID', [ 0;],'showRaw', [ 0;],'showRawMsg', [ 0;],'useStartVals', [ 0;],'extendedId', [ 0;],'showAge', [ 1;],'useSimFunc', [ 0;],'sim_func_name', '''''','fill', [ 0;],'editID', [ 0;],'signalOrder', [ 1;],'signalAscDes', [ 1;],'msgLength', [ 8;])  canBus='CAN2'  mailbox=''  payloadMask=[]  payloadValue=[]  idMask=hex2dec('1FFFFFFF')  queueSize=1  showID=0  label=1  fill=0  id=165  showRaw=0  showAge=1  signalOrder=1  signalInfo={{struct('Name', 'PM_motorSpeed','StartBit', [ 16;],'SignalSize', [ 16;],'ByteOrder', 'LittleEndian','ValueType', 'SIGNED','Class', 'int16','Signed', [ 1;],'Factor', [ 1;],'Offset', [ 0;],'Min', [ -32768;],'Max', [ 32767;],'Units', 'rpm','StartVal', [ 0;],'Comment', 'The measured speed of the motor','Multiplexed', [ 0;],'Multiplexor', [ 0;],'MultiplexMode_Min', [ 0;],'MultiplexMode_Max', [ 0;]),struct('Name', 'PM_electricalOutputFrequency','StartBit', [ 32;],'SignalSize', [ 16;],'ByteOrder', 'LittleEndian','ValueType', 'SIGNED','Class', 'int16','Signed', [ 1;],'Factor', [ 0.1;],'Offset', [ 0;],'Min', [ -3276.8;],'Max', [ 3276.7;],'Units', 'Hz','StartVal', [ 0;],'Comment', 'The actual frequency of the inverter','Multiplexed', [ 0;],'Multiplexor', [ 0;],'MultiplexMode_Min', [ 0;],'MultiplexMode_Max', [ 0;]),struct('Name', 'PM_electricalMotorAngle','StartBit', [ 0;],'SignalSize', [ 16;],'ByteOrder', 'LittleEndian','ValueType', 'UNSIGNED','Class', 'uint16','Signed', [ 0;],'Factor', [ 0.1;],'Offset', [ 0;],'Min', [ 0;],'Max', [ 6553.5;],'Units', 'deg','StartVal', [ 0;],'Comment', 'The Electrical Angle of the motor as read by the encoder or resolver','Multiplexed', [ 0;],'Multiplexor', [ 0;],'MultiplexMode_Min', [ 0;],'MultiplexMode_Max', [ 0;]),struct('Name', 'PM_deltaResolverFiltered','StartBit', [ 48;],'SignalSize', [ 16;],'ByteOrder', 'LittleEndian','ValueType', 'SIGNED','Class', 'int16','Signed', [ 1;],'Factor', [ 0.1;],'Offset', [ 0;],'Min', [ -3276.8;],'Max', [ 3276.7;],'Units', 'deg','StartVal', [ 0;],'Comment', 'Used in calibration of resolver angle adjustment','Multiplexed', [ 0;],'Multiplexor', [ 0;],'MultiplexMode_Min', [ 0;],'MultiplexMode_Max', [ 0;])}}  showRawMsg=0  useSimFunc=0  sim_func_name=''  useStartVals=0  extendedId=0
      settings: SourceProductName=Raptor
  raptor_can_rxmsg7 : Raptor_lib/CAN/raptor_can_rxmsg  canDefinition=struct('dbcFile', 'raptor_CAN2.dbc','message', 'PM_166','comment', '','signals', {{'PM_dcBusCurrent','PM_phaseACurrent','PM_phaseBCurrent','PM_phaseCCurrent'}},'enabled', [ 1 1 1 1;],'scaled', [ 1 1 1 1;],'canBus', '''CAN2''','messageID', [ 166;],'idMask', [ 536870911;],'payloadMask', [],'payloadValue', [],'period', [ 0;],'mailbox', '''''','queueSize', [ 1;],'label', [ 1;],'ver', [ 2;],'showID', [ 0;],'showRaw', [ 0;],'showRawMsg', [ 0;],'useStartVals', [ 0;],'extendedId', [ 0;],'showAge', [ 1;],'useSimFunc', [ 0;],'sim_func_name', '''''','fill', [ 0;],'editID', [ 0;],'signalOrder', [ 1;],'signalAscDes', [ 1;],'msgLength', [ 8;])  canBus='CAN2'  mailbox=''  payloadMask=[]  payloadValue=[]  idMask=hex2dec('1FFFFFFF')  queueSize=1  showID=0  label=1  fill=0  id=166  showRaw=0  showAge=1  signalOrder=1  signalInfo={{struct('Name', 'PM_phaseCCurrent','StartBit', [ 32;],'SignalSize', [ 16;],'ByteOrder', 'LittleEndian','ValueType', 'SIGNED','Class', 'int16','Signed', [ 1;],'Factor', [ 0.1;],'Offset', [ 0;],'Min', [ -3276.8;],'Max', [ 3276.7;],'Units', 'A','StartVal', [ 0;],'Comment', 'The measured value of Phase C current','Multiplexed', [ 0;],'Multiplexor', [ 0;],'MultiplexMode_Min', [ 0;],'MultiplexMode_Max', [ 0;]),struct('Name', 'PM_phaseBCurrent','StartBit', [ 16;],'SignalSize', [ 16;],'ByteOrder', 'LittleEndian','ValueType', 'SIGNED','Class', 'int16','Signed', [ 1;],'Factor', [ 0.1;],'Offset', [ 0;],'Min', [ -3276.8;],'Max', [ 3276.7;],'Units', 'A','StartVal', [ 0;],'Comment', 'The measured value of Phase B current','Multiplexed', [ 0;],'Multiplexor', [ 0;],'MultiplexMode_Min', [ 0;],'MultiplexMode_Max', [ 0;]),struct('Name', 'PM_phaseACurrent','StartBit', [ 0;],'SignalSize', [ 16;],'ByteOrder', 'LittleEndian','ValueType', 'SIGNED','Class', 'int16','Signed', [ 1;],'Factor', [ 0.1;],'Offset', [ 0;],'Min', [ -3276.8;],'Max', [ 3276.7;],'Units', 'A','StartVal', [ 0;],'Comment', 'The measured value of Phase A current','Multiplexed', [ 0;],'Multiplexor', [ 0;],'MultiplexMode_Min', [ 0;],'MultiplexMode_Max', [ 0;]),struct('Name', 'PM_dcBusCurrent','StartBit', [ 48;],'SignalSize', [ 16;],'ByteOrder', 'LittleEndian','ValueType', 'SIGNED','Class', 'int16','Signed', [ 1;],'Factor', [ 0.1;],'Offset', [ 0;],'Min', [ -3276.8;],'Max', [ 3276.7;],'Units', 'A','StartVal', [ 0;],'Comment', 'The calculated DC Bus Current','Multiplexed', [ 0;],'Multiplexor', [ 0;],'MultiplexMode_Min', [ 0;],'MultiplexMode_Max', [ 0;])}}  showRawMsg=0  useSimFunc=0  sim_func_name=''  useStartVals=0  extendedId=0
      settings: SourceProductName=Raptor
  raptor_can_rxmsg8 : Raptor_lib/CAN/raptor_can_rxmsg  canDefinition=struct('dbcFile', 'raptor_CAN2.dbc','message', 'PM_167','comment', '','signals', {{'PM_dcBusVolt','PM_outputVolt','PM_vabVdVolt','PM_vbcVqVolt'}},'enabled', [ 1 1 1 1;],'scaled', [ 1 1 1 1;],'canBus', '''CAN2''','messageID', [ 167;],'idMask', [ 536870911;],'payloadMask', [],'payloadValue', [],'period', [ 0;],'mailbox', '''''','queueSize', [ 1;],'label', [ 1;],'ver', [ 2;],'showID', [ 0;],'showRaw', [ 0;],'showRawMsg', [ 0;],'useStartVals', [ 0;],'extendedId', [ 0;],'showAge', [ 1;],'useSimFunc', [ 0;],'sim_func_name', '''''','fill', [ 0;],'editID', [ 0;],'signalOrder', [ 1;],'signalAscDes', [ 1;],'msgLength', [ 8;])  canBus='CAN2'  mailbox=''  payloadMask=[]  payloadValue=[]  idMask=hex2dec('1FFFFFFF')  queueSize=1  showID=0  label=1  fill=0  id=167  showRaw=0  showAge=1  signalOrder=1  signalInfo={{struct('Name', 'PM_vbcVqVolt','StartBit', [ 48;],'SignalSize', [ 16;],'ByteOrder', 'LittleEndian','ValueType', 'SIGNED','Class', 'int16','Signed', [ 1;],'Factor', [ 0.1;],'Offset', [ 0;],'Min', [ -3276.8;],'Max', [ 3276.7;],'Units', 'V','StartVal', [ 0;],'Comment', 'Measured value of the voltage between Phase B and Phase C','Multiplexed', [ 0;],'Multiplexor', [ 0;],'MultiplexMode_Min', [ 0;],'MultiplexMode_Max', [ 0;]),struct('Name', 'PM_vabVdVolt','StartBit', [ 32;],'SignalSize', [ 16;],'ByteOrder', 'LittleEndian','ValueType', 'SIGNED','Class', 'int16','Signed', [ 1;],'Factor', [ 0.1;],'Offset', [ 0;],'Min', [ -3276.8;],'Max', [ 3276.7;],'Units', 'V','StartVal', [ 0;],'Comment', 'Measured value of the voltage between Phase A and Phase B','Multiplexed', [ 0;],'Multiplexor', [ 0;],'MultiplexMode_Min', [ 0;],'MultiplexMode_Max', [ 0;]),struct('Name', 'PM_outputVolt','StartBit', [ 16;],'SignalSize', [ 16;],'ByteOrder', 'LittleEndian','ValueType', 'SIGNED','Class', 'int16','Signed', [ 1;],'Factor', [ 0.1;],'Offset', [ 0;],'Min', [ -3276.8;],'Max', [ 3276.7;],'Units', 'V','StartVal', [ 0;],'Comment', 'The calculated value of the output voltage, in peak line-neutral volts','Multiplexed', [ 0;],'Multiplexor', [ 0;],'MultiplexMode_Min', [ 0;],'MultiplexMode_Max', [ 0;]),struct('Name', 'PM_dcBusVolt','StartBit', [ 0;],'SignalSize', [ 16;],'ByteOrder', 'LittleEndian','ValueType', 'SIGNED','Class', 'int16','Signed', [ 1;],'Factor', [ 0.1;],'Offset', [ 0;],'Min', [ -3276.8;],'Max', [ 3276.7;],'Units', 'V','StartVal', [ 0;],'Comment', 'The actual measured value of the DC bus voltage','Multiplexed', [ 0;],'Multiplexor', [ 0;],'MultiplexMode_Min', [ 0;],'MultiplexMode_Max', [ 0;])}}  showRawMsg=0  useSimFunc=0  sim_func_name=''  useStartVals=0  extendedId=0
      settings: SourceProductName=Raptor
  raptor_can_rxmsg9 : Raptor_lib/CAN/raptor_can_rxmsg  canDefinition=struct('dbcFile', 'raptor_CAN2.dbc','message', 'PM_168','comment', '','signals', {{'PM_fluxCommand','PM_fluxFeedback','PM_id','PM_iq'}},'enabled', [ 1 1 1 1;],'scaled', [ 1 1 1 1;],'canBus', '''CAN2''','messageID', [ 168;],'idMask', [ 536870911;],'payloadMask', [],'payloadValue', [],'period', [ 0;],'mailbox', '''''','queueSize', [ 1;],'label', [ 1;],'ver', [ 2;],'showID', [ 0;],'showRaw', [ 0;],'showRawMsg', [ 0;],'useStartVals', [ 0;],'extendedId', [ 0;],'showAge', [ 1;],'useSimFunc', [ 0;],'sim_func_name', '''''','fill', [ 0;],'editID', [ 0;],'signalOrder', [ 1;],'signalAscDes', [ 1;],'msgLength', [ 8;])  canBus='CAN2'  mailbox=''  payloadMask=[]  payloadValue=[]  idMask=hex2dec('1FFFFFFF')  queueSize=1  showID=0  label=1  fill=0  id=168  showRaw=0  showAge=1  signalOrder=1  signalInfo={{struct('Name', 'PM_iq','StartBit', [ 48;],'SignalSize', [ 16;],'ByteOrder', 'LittleEndian','ValueType', 'SIGNED','Class', 'int16','Signed', [ 1;],'Factor', [ 0.1;],'Offset', [ 0;],'Min', [ -3276.8;],'Max', [ 3276.7;],'Units', 'A','StartVal', [ 0;],'Comment', 'The measured Iq current','Multiplexed', [ 0;],'Multiplexor', [ 0;],'MultiplexMode_Min', [ 0;],'MultiplexMode_Max', [ 0;]),struct('Name', 'PM_id','StartBit', [ 32;],'SignalSize', [ 16;],'ByteOrder', 'LittleEndian','ValueType', 'SIGNED','Class', 'int16','Signed', [ 1;],'Factor', [ 0.1;],'Offset', [ 0;],'Min', [ -3276.8;],'Max', [ 3276.7;],'Units', 'A','StartVal', [ 0;],'Comment', 'The measured Id current','Multiplexed', [ 0;],'Multiplexor', [ 0;],'MultiplexMode_Min', [ 0;],'MultiplexMode_Max', [ 0;]),struct('Name', 'PM_fluxFeedback','StartBit', [ 16;],'SignalSize', [ 16;],'ByteOrder', 'LittleEndian','ValueType', 'SIGNED','Class', 'int16','Signed', [ 1;],'Factor', [ 0.001;],'Offset', [ 0;],'Min', [ -32.768;],'Max', [ 32.767;],'Units', 'Wb','StartVal', [ 0;],'Comment', 'The estimated flux','Multiplexed', [ 0;],'Multiplexor', [ 0;],'MultiplexMode_Min', [ 0;],'MultiplexMode_Max', [ 0;]),struct('Name', 'PM_fluxCommand','StartBit', [ 0;],'SignalSize', [ 16;],'ByteOrder', 'LittleEndian','ValueType', 'SIGNED','Class', 'int16','Signed', [ 1;],'Factor', [ 0.001;],'Offset', [ 0;],'Min', [ -32.768;],'Max', [ 32.767;],'Units', 'Wb','StartVal', [ 0;],'Comment', 'The commanded flux','Multiplexed', [ 0;],'Multiplexor', [ 0;],'MultiplexMode_Min', [ 0;],'MultiplexMode_Max', [ 0;])}}  showRawMsg=0  useSimFunc=0  sim_func_name=''  useStartVals=0  extendedId=0
      settings: SourceProductName=Raptor
  CAN1_pm_bus : Outport
  CAN2_pm_bus : Outport  Port=2
  wires:
  raptor_can_rxmsg19/1 -> Bus Creator/1  "Age"
  raptor_can_rxmsg19/2 -> Bus Creator/2  "PM_bmsActive"
  raptor_can_rxmsg19/3 -> Bus Creator/3  "PM_bmsTorqueLimiting"
  raptor_can_rxmsg19/4 -> Bus Creator/4  "PM_counterMsg170"
  raptor_can_rxmsg19/5 -> Bus Creator/5  "PM_directionCommand"
  raptor_can_rxmsg19/6 -> Bus Creator/6  "PM_inverterCommandMode"
  raptor_can_rxmsg19/7 -> Bus Creator/7  "PM_inverterDischargeMode"
  raptor_can_rxmsg19/8 -> Bus Creator/8  "PM_inverterEnableLockout"
  raptor_can_rxmsg19/9 -> Bus Creator/9  "PM_inverterEnableState"
  raptor_can_rxmsg19/10 -> Bus Creator/10  "PM_inverterRunMode"
  raptor_can_rxmsg19/11 -> Bus Creator/11  "PM_inverterState"
  raptor_can_rxmsg19/12 -> Bus Creator/12  "PM_lowSpeedLimiting"
  raptor_can_rxmsg19/13 -> Bus Creator/13  "PM_maxSpeedLimiting"
  raptor_can_rxmsg19/14 -> Bus Creator/14  "PM_pwmFrequency"
  raptor_can_rxmsg19/15 -> Bus Creator/15  "PM_relayStatus1"
  raptor_can_rxmsg19/16 -> Bus Creator/16  "PM_relayStatus2"
  raptor_can_rxmsg19/17 -> Bus Creator/17  "PM_relayStatus3"
  raptor_can_rxmsg19/18 -> Bus Creator/18  "PM_relayStatus4"
  raptor_can_rxmsg19/19 -> Bus Creator/19  "PM_relayStatus5"
  raptor_can_rxmsg19/20 -> Bus Creator/20  "PM_relayStatus6"
  raptor_can_rxmsg19/21 -> Bus Creator/21  "PM_startModeActive"
  raptor_can_rxmsg19/22 -> Bus Creator/22  "PM_vsmState"
  Bus Creator/1 -> Bus Creator19/1  "CAN1_pm_170_bus"
  raptor_can_rxmsg2/3 -> Bus Creator1/3  "PM_moduleATemp"
  raptor_can_rxmsg2/4 -> Bus Creator1/4  "PM_moduleBTemp"
  raptor_can_rxmsg2/5 -> Bus Creator1/5  "PM_moduleCTemp"
  raptor_can_rxmsg2/2 -> Bus Creator1/2  "PM_gateDriverBoard"
  raptor_can_rxmsg2/1 -> Bus Creator1/1  "Age"
  raptor_can_rxmsg1/4 -> Bus Creator2/4  "PM_rtd2Temp"
  raptor_can_rxmsg1/5 -> Bus Creator2/5  "PM_rtd3Temp"
  raptor_can_rxmsg1/3 -> Bus Creator2/3  "PM_rtd1Temp"
  raptor_can_rxmsg1/2 -> Bus Creator2/2  "PM_controlBoardTemp"
  raptor_can_rxmsg1/1 -> Bus Creator2/1  "Age"
  raptor_can_rxmsg3/2 -> Bus Creator3/2  "PM_motorTemp"
  raptor_can_rxmsg3/1 -> Bus Creator3/1  "Age"
  raptor_can_rxmsg3/3 -> Bus Creator3/3  "PM_rtd4Temp"
  raptor_can_rxmsg3/4 -> Bus Creator3/4  "PM_rtd5Temp"
  raptor_can_rxmsg3/5 -> Bus Creator3/5  "PM_torqueShudder"
  raptor_can_rxmsg4/1 -> Bus Creator4/1  "Age"
  raptor_can_rxmsg4/2 -> Bus Creator4/2  "PM_analogInputVolt1"
  raptor_can_rxmsg4/3 -> Bus Creator4/3  "PM_analogInputVolt2"
  raptor_can_rxmsg4/4 -> Bus Creator4/4  "PM_analogInputVolt3"
  raptor_can_rxmsg4/5 -> Bus Creator4/5  "PM_analogInputVolt4"
  raptor_can_rxmsg4/6 -> Bus Creator4/6  "PM_analogInputVolt5"
  raptor_can_rxmsg4/7 -> Bus Creator4/7  "PM_analogInputVolt6"
  raptor_can_rxmsg5/1 -> Bus Creator5/1  "Age"
  raptor_can_rxmsg5/2 -> Bus Creator5/2  "PM_digitalInputStatus1"
  raptor_can_rxmsg5/3 -> Bus Creator5/3  "PM_digitalInputStatus2"
  raptor_can_rxmsg5/4 -> Bus Creator5/4  "PM_digitalInputStatus3"
  raptor_can_rxmsg5/5 -> Bus Creator5/5  "PM_digitalInputStatus4"
  raptor_can_rxmsg5/6 -> Bus Creator5/6  "PM_digitalInputStatus5"
  raptor_can_rxmsg5/7 -> Bus Creator5/7  "PM_digitalInputStatus6"
  raptor_can_rxmsg5/8 -> Bus Creator5/8  "PM_digitalInputStatus7"
  raptor_can_rxmsg5/9 -> Bus Creator5/9  "PM_digitalInputStatus8"
  raptor_can_rxmsg6/1 -> Bus Creator6/1  "Age"
  raptor_can_rxmsg6/2 -> Bus Creator6/2  "PM_deltaResolverFiltered"
  raptor_can_rxmsg6/3 -> Bus Creator6/3  "PM_electricalMotorAngle"
  raptor_can_rxmsg6/4 -> Bus Creator6/4  "PM_electricalOutputFrequency"
  raptor_can_rxmsg6/5 -> Bus Creator6/5  "PM_motorSpeed"
  raptor_can_rxmsg7/1 -> Bus Creator7/1  "Age"
  raptor_can_rxmsg7/2 -> Bus Creator7/2  "PM_dcBusCurrent"
  raptor_can_rxmsg7/3 -> Bus Creator7/3  "PM_phaseACurrent"
  raptor_can_rxmsg7/4 -> Bus Creator7/4  "PM_phaseBCurrent"
  raptor_can_rxmsg7/5 -> Bus Creator7/5  "PM_phaseCCurrent"
  raptor_can_rxmsg8/1 -> Bus Creator8/1  "Age"
  raptor_can_rxmsg8/2 -> Bus Creator8/2  "PM_dcBusVolt"
  raptor_can_rxmsg8/3 -> Bus Creator8/3  "PM_outputVolt"
  raptor_can_rxmsg8/4 -> Bus Creator8/4  "PM_vabVdVolt"
  raptor_can_rxmsg8/5 -> Bus Creator8/5  "PM_vbcVqVolt"
  raptor_can_rxmsg9/1 -> Bus Creator9/1  "Age"
  raptor_can_rxmsg9/2 -> Bus Creator9/2  "PM_fluxCommand"
  raptor_can_rxmsg9/3 -> Bus Creator9/3  "PM_fluxFeedback"
  raptor_can_rxmsg9/4 -> Bus Creator9/4  "PM_id"
  raptor_can_rxmsg9/5 -> Bus Creator9/5  "PM_iq"
  raptor_can_rxmsg10/1 -> Bus Creator10/1  "Age"
  raptor_can_rxmsg10/2 -> Bus Creator10/2  "PM_refVolt120"
  raptor_can_rxmsg10/3 -> Bus Creator10/3  "PM_refVolt15"
  raptor_can_rxmsg10/4 -> Bus Creator10/4  "PM_refVolt25"
  raptor_can_rxmsg10/5 -> Bus Creator10/5  "PM_refVolt50"
  raptor_can_rxmsg11/1 -> Bus Creator11/1  "Age"
  raptor_can_rxmsg11/2 -> Bus Creator11/2  "PM_postFaultHi"
  raptor_can_rxmsg11/3 -> Bus Creator11/3  "PM_postFaultLo"
  raptor_can_rxmsg11/4 -> Bus Creator11/4  "PM_runFaultHi"
  raptor_can_rxmsg11/5 -> Bus Creator11/5  "PM_runFaultLo"
  raptor_can_rxmsg12/1 -> Bus Creator12/1  "Age"
  raptor_can_rxmsg12/2 -> Bus Creator12/2  "PM_commandedTorque"
  raptor_can_rxmsg12/3 -> Bus Creator12/3  "PM_powerOnTimer"
  raptor_can_rxmsg12/4 -> Bus Creator12/4  "PM_torqueFeedback"
  raptor_can_rxmsg13/1 -> Bus Creator13/1  "Age"
  raptor_can_rxmsg13/2 -> Bus Creator13/2  "PM_fluxWeakeningOutput"
  raptor_can_rxmsg13/3 -> Bus Creator13/3  "PM_idCommand"
  raptor_can_rxmsg13/4 -> Bus Creator13/4  "PM_iqCommand"
  raptor_can_rxmsg13/5 -> Bus Creator13/5  "PM_modulationIndex"
  raptor_can_rxmsg14/1 -> Bus Creator14/1  "Age"
  raptor_can_rxmsg14/2 -> Bus Creator14/2  "PM_datecodeMMDD"
  raptor_can_rxmsg14/3 -> Bus Creator14/3  "PM_datecodeYYYY"
  raptor_can_rxmsg14/4 -> Bus Creator14/4  "PM_projectCodeEEPVer"
  raptor_can_rxmsg14/5 -> Bus Creator14/5  "PM_swVersion"
  raptor_can_rxmsg15/1 -> Bus Creator15/1  "Age"
  raptor_can_rxmsg15/2 -> Bus Creator15/2  "PM_bufferRecord"
  raptor_can_rxmsg15/3 -> Bus Creator15/3  "PM_bufferSegment"
  raptor_can_rxmsg15/4 -> Bus Creator15/4  "PM_diagData1"
  raptor_can_rxmsg15/5 -> Bus Creator15/5  "PM_diagData2"
  raptor_can_rxmsg15/6 -> Bus Creator15/6  "PM_diagData3"
  raptor_can_rxmsg16/1 -> Bus Creator16/1  "Age"
  raptor_can_rxmsg16/2 -> Bus Creator16/2  "PM_fastDCBusVolt"
  raptor_can_rxmsg16/3 -> Bus Creator16/3  "PM_fastMotorSpeed"
  raptor_can_rxmsg16/4 -> Bus Creator16/4  "PM_fastTorqueCommand"
  raptor_can_rxmsg16/5 -> Bus Creator16/5  "PM_fastTorqueFeedback"
  raptor_can_rxmsg17/1 -> Bus Creator17/1  "Age"
  raptor_can_rxmsg17/2 -> Bus Creator17/2  "PM_dataCommand"
  raptor_can_rxmsg17/3 -> Bus Creator17/3  "PM_parameterAddressCommand"
  raptor_can_rxmsg17/4 -> Bus Creator17/4  "PM_readWriteCommand"
  raptor_can_rxmsg18/2 -> Bus Creator18/2  "PM_dataResponse"
  raptor_can_rxmsg18/1 -> Bus Creator18/1  "Age"
  raptor_can_rxmsg18/3 -> Bus Creator18/3  "PM_parameterAddressResponse"
  raptor_can_rxmsg18/4 -> Bus Creator18/4  "PM_writeSuccess"
  Bus Creator2/1 -> Bus Creator20/2  "CAN2_pm_161_bus"
  Bus Creator3/1 -> Bus Creator20/3  "CAN2_pm_162_bus"
  Bus Creator4/1 -> Bus Creator20/4  "CAN2_pm_163_bus"
  Bus Creator5/1 -> Bus Creator20/5  "CAN2_pm_164_bus"
  Bus Creator6/1 -> Bus Creator20/6  "CAN2_pm_165_bus"
  Bus Creator8/1 -> Bus Creator20/8  "CAN2_pm_167_bus"
  Bus Creator9/1 -> Bus Creator20/9  "CAN2_pm_168_bus"
  Bus Creator10/1 -> Bus Creator20/10  "CAN2_pm_169_bus"
  Bus Creator11/1 -> Bus Creator20/11  "CAN2_pm_171_bus"
  Bus Creator12/1 -> Bus Creator20/12  "CAN2_pm_172_bus"
  Bus Creator13/1 -> Bus Creator20/13  "CAN2_pm_173_bus"
  Bus Creator14/1 -> Bus Creator20/14  "CAN2_pm_174_bus"
  Bus Creator15/1 -> Bus Creator20/15  "CAN2_pm_175_bus"
  Bus Creator16/1 -> Bus Creator20/16  "CAN2_pm_176_bus"
  Bus Creator17/1 -> Bus Creator20/17  "CAN2_pm_193_bus"
  Bus Creator18/1 -> Bus Creator20/18  "CAN2_pm_194_bus"
  Bus Creator19/1 -> CAN1_pm_bus/1  "CAN1_pm_bus"
  Bus Creator1/1 -> Bus Creator20/1  "CAN2_pm_160_bus"
  Bus Creator7/1 -> Bus Creator20/7  "CAN2_pm_166_bus"
  Bus Creator20/1 -> CAN2_pm_bus/1  "CAN2_pm_bus"
